simulink model "Simple_PID_Controller"  (R2024b)
settings: Solver=VariableStepAuto  StartTime=0.0  StopTime=20  RelTol=1e-3
settings Model: Creator=User  LastModifiedBy=User

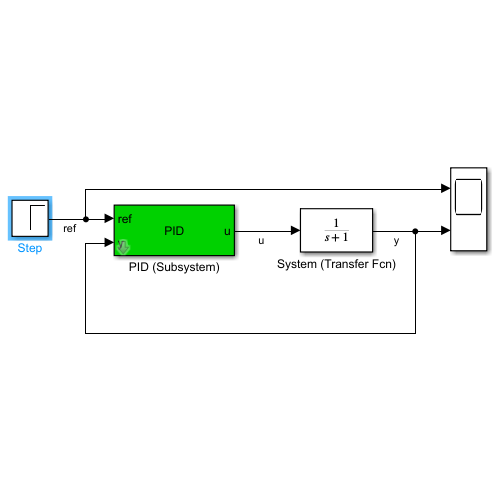
[thumbnail: Simulink's stored preview of the top-level diagram]
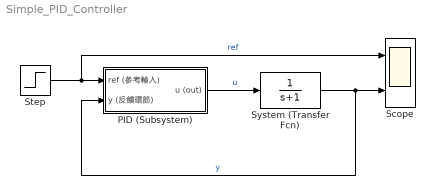
== system Simple_PID_Controller ==
  PID (Subsystem) : Subsystem  mask{KP=3, KI=1, KD=1}
      mask prompts: KP "value-KP"; KI "value-KI"; KD "value-KD"
      mask Display:
      | % 此為創建 [簡易 PID 控制器] 的變數遮罩，用於快速變數設值
      | 
      | % 步驟
      | % 1.在此的 Icon 區，加入以下內容於此。
      | % 2.在此的 Parameters & Dialog 區，新增 3 個 Edit，和設值。
      | 
      | disp('PID') % 模塊名稱
      | port_label('input',1,'ref') % 輸入接口標籤，輸入參考
      | port_label('input',2,'y') % 輸入接口標籤，傳回值
      | port_label('output',1,'u') % 輸出接口標籤，輸出
  Scope : Scope  NumInputPorts=2
  Step : Step  Time=0  SampleTime=0
  System (Transfer Fcn) : TransferFcn  Denominator=[1 1]
  wires:
  Step/1 -> Scope/1, PID (Subsystem)/1(ref (參考輸入))  "ref"
  PID (Subsystem)/1(u (out)) -> System (Transfer Fcn)/1  "u"
  System (Transfer Fcn)/1 -> Scope/2, PID (Subsystem)/2(y (反饋環節))  "y"

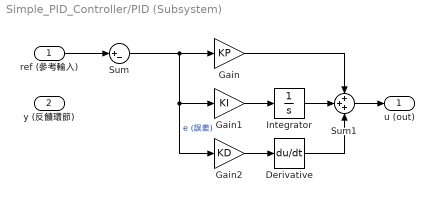
== system Simple_PID_Controller/PID (Subsystem) ==
  ref (參考輸入) : Inport
  y (反饋環節) : Inport  Port=2
  Derivative : Derivative
  Gain : Gain  Gain=KP
  Gain1 : Gain  Gain=KI
  Gain2 : Gain  Gain=KD
  Integrator : Integrator
  Sum : Sum  Inputs=|+-
  Sum1 : Sum  Inputs=+++
  u (out) : Outport
  wires:
  ref (參考輸入)/1 -> Sum/1
  Sum/1 -> Gain2/1, Gain1/1, Gain/1  "e (誤差)"
  Gain/1 -> Sum1/1
  Sum1/1 -> u (out)/1
  Gain1/1 -> Integrator/1
  Integrator/1 -> Sum1/2
  Gain2/1 -> Derivative/1
  Derivative/1 -> Sum1/3
